simulink model "LCL_Inverter_Template"  (R2017a)
settings: Solver=ode4  StartTime=0.0  StopTime=0.04  FixedStep=1e-7  MaxStep=1e-7  AbsTol=1e-9
InitFcn:
  | clc;
  | clear all;
  | 
  | Ts_Control = 1e-4;
  | Ts_Pw = 1e-7;
  | T_dead = 30 * Ts_Pw;
  | 
  | fg=50;
  | Ed=360;
  | 
  | Kd = 0.12 ;
  | 
  | Kp = 0.067 ;
  | Ki = 330 ;
  | 
  | Apt_Carrier = 3 ;
  | 
  | C = 10e-6;
  | R =  0.05 ;
  | L1 = 600e-6 ;
  | R1 =  0.05 ;
  | L2 = 150e-6 ;
  | R2 =  0.05 ;
undefined symbols (not defined in the file or in its folder): DiscIntNeverNeededParam
libraries: powerlib x12, simulink x3, powerlib_extras x2, powerlib_meascontrol x2
settings Model: Creator=Administrator  LastModifiedBy=donghao
settings SolverCC: ZeroCrossControl=DisableAll
settings DataIOCC: LimitDataPoints=on  SaveFormat=Array  SignalLoggingSaveFormat=ModelDataLogs
settings OptimizationCC: ExpressionDepthLimit=2147483647  InitFltsAndDblsToZero=on  LifeSpan=inf
settings DebuggingCC: SaveWithParameterizedLinksMsg=none  UnderspecifiedInitializationDetection=Classic  MergeDetectMultiDrivingBlocksExec=none  SignalResolutionControl=TryResolveAllWithWarning  SolverPrmCheckMsg=warning  MultiTaskDSMMsg=warning  MultiTaskCondExecSysMsg=none  FcnCallInpInsideContextMsg=warning  UnconnectedInputMsg=none  UnconnectedOutputMsg=none  UnconnectedLineMsg=none  AllowSymbolicDim=off  StateNameClashWarn=warning  SFUnexpectedBacktrackingDiag=warning  SFNoUnconditionalDefaultTransitionDiag=warning  SFExecutionAtInitializationDiag=none
settings HardwareCC: ProdBitPerPointer=32  ProdBitPerSizeT=32  ProdBitPerPtrDiffT=32  ProdLargestAtomicFloat=None  ProdIntDivRoundTo=Undefined  ProdEndianess=Unspecified  ProdWordSize=32  ProdHWDeviceType=32-bit Generic
settings ModelReferenceCC: PropagateSignalLabelsOutOfModel=off
settings SFSimCC: SimParseCustomCode=off
settings GRTTargetCC: TargetFcnLib=ansi_tfl_tmw.mat  TargetLangStandard=C89/C90 (ANSI)  GeneratePreprocessorConditionals=Disable all  CombineOutputUpdateFcns=off  GRTInterface=on
settings ConfigComp: CovMetricSettings=dw  CovHtmlReporting=on  CovSaveCumulativeToWorkspaceVar=on  CovSaveSingleToWorkspaceVar=on  CovExternalEMLEnable=off

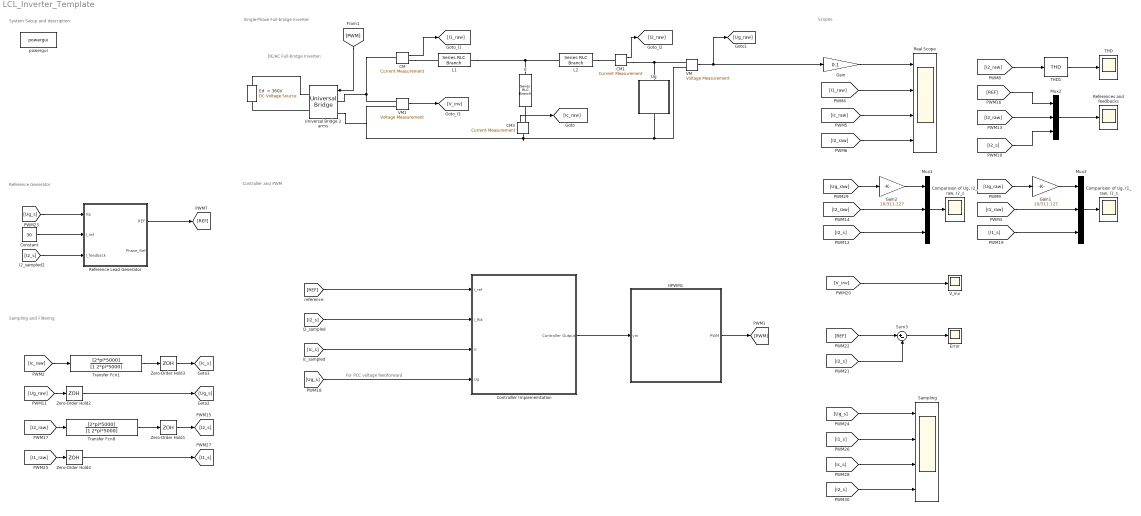
== system LCL_Inverter_Template ==
  note: For PCC voltage feedforward
  note: Sampling and Filtering
  note: System Setup and description:
  note: Single-Phase Full-bridge Inverter
  note: Scopes
  note: Controller and PWM
  note: DC/AC Full-bridge Inverter:
  note: Reference Generator
  C : powerlib/Elements/Series RLC Branch  LConnTagsString=__new0  RConnTagsString=__new0  BranchType=RC  Resistance=R  Inductance=0  SetiL0=off  InitialCurrent=0  Capacitance=C  Setx0=off  InitialVoltage=0  Measurements=None
  CM : powerlib/Measurements/Current Measurement  PhasorSimulation=off  OutputType=Complex  PSBequivalent=0
  CM1 : powerlib/Measurements/Current Measurement  PhasorSimulation=off  OutputType=Complex  PSBequivalent=0
  CM3 : powerlib/Measurements/Current Measurement  PhasorSimulation=off  OutputType=Complex  PSBequivalent=0
  "Comparision of Ug, I1_raw, I1_s" : Scope
  "Comparision of Ug, I2_raw, I2_s" : Scope
  Constant : Constant  Value=30
  Controlller Implememtation : Subsystem
  "Ed  = 360V  " : powerlib/Electrical Sources/DC Voltage Source  Description=source block  Amplitude=Ed  Measurements=None
      settings: AttributesFormatString=\n
  Error : Scope
  Gain : Gain  Gain=0.1
  Gain1 : Gain  Gain=10/311.127
  Gain2 : Gain  Gain=10/311.127
  HPWM1 : Subsystem
  L1 : powerlib/Elements/Series RLC Branch  LConnTagsString=__new0  RConnTagsString=__new0  BranchType=RL  Resistance=R1  Inductance=L1  SetiL0=off  InitialCurrent=0  Capacitance=1e-6  Setx0=off  InitialVoltage=0  Measurements=None
  L2 : powerlib/Elements/Series RLC Branch  LConnTagsString=__new0  RConnTagsString=__new0  BranchType=RL  Resistance=R2  Inductance=L2  SetiL0=off  InitialCurrent=0  Capacitance=1e-6  Setx0=off  InitialVoltage=0  Measurements=None
  Mux1 : Mux  Inputs=3
  Mux2 : Mux  Inputs=3
  Mux3 : Mux  Inputs=3
  Real Scope : Scope  NumInputPorts=4
  Reference Lead Generator : Subsystem
  References and feedbacks : Scope
  Sampling : Scope  NumInputPorts=4
  Sum3 : Sum  Inputs=|+-
  THD : Scope
  THD1 : powerlib_meascontrol/Measurements/THD  Freq=50  Ts=Ts_Pw
  Transfer Fcn1 : TransferFcn  Numerator=[2*pi*5000]  Denominator=[1 2*pi*5000]
  Transfer Fcn8 : TransferFcn  Numerator=[2*pi*5000]  Denominator=[1 2*pi*5000]
  Ug : Subsystem
  Universal Bridge 2 arms : powerlib/Power Electronics/Universal Bridge  Arms=2  SnubberResistance=1e3  SnubberCapacitance=1e-6  Device=IGBT / Diodes  Ron=1e-4  Lon=0  ForwardVoltages="[  1  1  ]"  ForwardVoltage=.8  GTOparameters=[ 10e-6 , 20e-6 ]  IGBTparameters=[ 1e-6 , 2e-6 ]  Measurements=None  Measurements_2=None  converterType=Rectifier
  VM : powerlib/Measurements/Voltage Measurement  PhasorSimulation=off  OutputType=Complex  PSBequivalent=0
  VM1 : powerlib/Measurements/Voltage Measurement  PhasorSimulation=off  OutputType=Complex  PSBequivalent=0
  V_inv : Scope
  Zero-Order Hold{1..4} (4 alike) : ZeroOrderHold  SampleTime=Ts_Control
  powergui : powerlib/powergui  SimulationMode=Discrete  SampleTime=Ts_Pw  frequency=60  Iterations=50  frequencyindice=50  Pbase=100e6  ErrMax=1e-4  UnitsV=kV  UnitsW=MW  buscounter=0  FunctionMessages=off  echomessages=off  EnableUseOfTLC=off  CurrentSourceSwitches=off  DisableSnubberDevices=off  DisableRonSwitches=off  DisableVfSwitches=off  DisplayEquations=off  SolverType=Tustin/Backward Euler (TBE)  Interpol=off  ExternalGateDelay=off  methode=off  Ts=0  x0status=blocks  SPID=off  SwTol=0  HookPort=off  RestoreLinks=warning  ResistiveCurrentMeasurement=off  Frange=[0:2:500]  Ylog=off  Xlog=on  ShowGrid=off  save=off  variable=ZData  structure=UGandIG1  ZoomFFT=off  StartTime=0.04  cycles=1  DisplayStyle=1  fundamental=50  FreqAxis=on  MaxFrequency=2000  frequencyindicesteady=1  RmsSteady=1  display=off
  wires:
  HPWM1/1(PWM) -> [PWM]
  VM/1 -> Gain/1, [Ug_raw]
  CM1/1 -> [I2_raw]
  Gain/1 -> Real Scope/1
  [I1_raw] -> Real Scope/2
  [Ic_raw] -> Real Scope/3
  [I2_raw] -> Real Scope/4
  Mux3/1 -> "Comparision of Ug, I1_raw, I1_s"/1
  [I1_raw] -> Mux3/2
  [Ug_raw] -> Gain1/1
  Gain1/1 -> Mux3/1
  [REF] -> Mux2/1
  Mux2/1 -> References and feedbacks/1
  [PWM] -> Universal Bridge 2 arms/1
  [I2_raw] -> THD1/1
  THD1/1 -> THD/1
  [I2_raw] -> Mux2/2
  CM3/1 -> [Ic_raw]
  CM/1 -> [I1_raw]
  Zero-Order Hold1/1 -> [I2_s]
  [I2_s] -> Controlller Implememtation/2(I_fbk)
  VM1/1 -> [V_inv]
  [V_inv] -> V_inv/1
  Reference Lead Generator/1(REF) -> [REF]
  [REF] -> Sum3/1
  [I2_s] -> Sum3/2
  Sum3/1 -> Error/1
  [Ug_s] -> Reference Lead Generator/1(Ug)
  [Ic_s] -> Controlller Implememtation/3(Ic)
  [Ug_s] -> Controlller Implememtation/4(Ug)
  Controlller Implememtation/1(Controller Output) -> HPWM1/1(vm)
  [Ug_raw] -> Zero-Order Hold2/1
  [REF] -> Controlller Implememtation/1(I_ref)
  Zero-Order Hold2/1 -> [Ug_s]
  Zero-Order Hold3/1 -> [Ic_s]
  [I2_s] -> Mux2/3
  [I1_s] -> Mux3/3
  [I1_raw] -> Zero-Order Hold4/1
  Zero-Order Hold4/1 -> [I1_s]
  [I2_s] -> Mux1/3
  [I2_raw] -> Mux1/2
  Gain2/1 -> Mux1/1
  [Ug_raw] -> Gain2/1
  Mux1/1 -> "Comparision of Ug, I2_raw, I2_s"/1
  [I2_s] -> Reference Lead Generator/3(I_feedback)
  Constant/1 -> Reference Lead Generator/2(I_ref)
  [I2_raw] -> Transfer Fcn8/1
  [Ug_s] -> Sampling/1
  [I1_s] -> Sampling/2
  [Ic_s] -> Sampling/3
  [I2_s] -> Sampling/4
  [Ic_raw] -> Transfer Fcn1/1
  Transfer Fcn8/1 -> Zero-Order Hold1/1
  Transfer Fcn1/1 -> Zero-Order Hold3/1
  connections:
  Universal Bridge 2 arms/RConn2 -- "Ed  = 360V  "/LConn1
  CM1/RConn1 -- VM/LConn1 -- Ug/RConn1
  L1/RConn1 -- L2/LConn1 -- C/LConn1
  CM/RConn1 -- L1/LConn1
  L2/RConn1 -- CM1/LConn1
  "Ed  = 360V  "/RConn1 -- Universal Bridge 2 arms/RConn1
  CM3/RConn1 -- C/RConn1
  VM1/LConn1 -- Universal Bridge 2 arms/LConn1 -- CM/LConn1
  Ug/LConn1 -- Universal Bridge 2 arms/LConn2 -- VM1/LConn2 -- CM3/LConn1 -- VM/LConn2

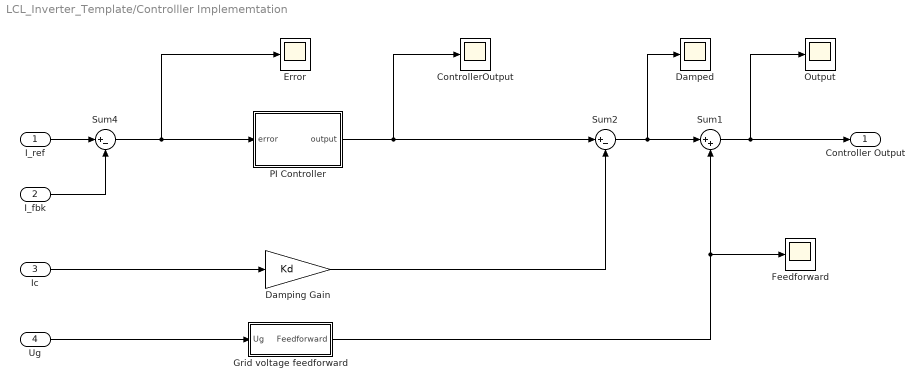
== system LCL_Inverter_Template/Controlller Implememtation ==
  I_ref : Inport
  I_fbk : Inport  Port=2
  Ic : Inport  Port=3
  Ug : Inport  Port=4
  ControllerOutput : Scope
  Damped : Scope
  Damping Gain : Gain  Gain=Kd
  Error : Scope
  Feedforward : Scope
  Grid voltage feedforward : Subsystem
  Output : Scope
  PI Controller : Subsystem
  Sum1 : Sum  Inputs=|++
  Sum2 : Sum  Inputs=|+-
  Sum4 : Sum  Inputs=|+-
  Controller Output : Outport
  wires:
  Ug/1 -> Grid voltage feedforward/1(Ug)
  Ic/1 -> Damping Gain/1
  PI Controller/1(output) -> Sum2/1, ControllerOutput/1
  Grid voltage feedforward/1(Feedforward) -> Feedforward/1, Sum1/2
  Sum1/1 -> Controller Output/1, Output/1
  Sum2/1 -> Sum1/1, Damped/1
  I_ref/1 -> Sum4/1
  I_fbk/1 -> Sum4/2
  Sum4/1 -> Error/1, PI Controller/1(error)
  Damping Gain/1 -> Sum2/2

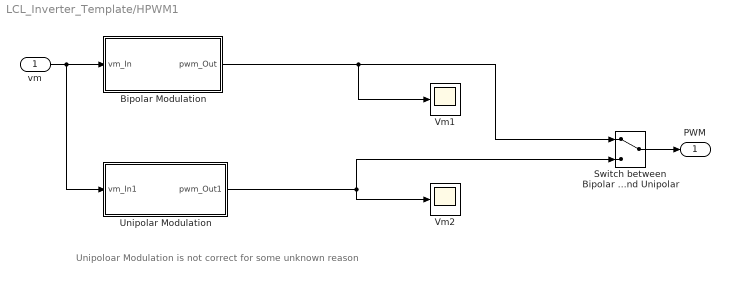
== system LCL_Inverter_Template/HPWM1 ==
  note: Unipoloar Modulation is not correct for some unknown reason
  vm : Inport
  Bipolar Modulation : Subsystem
  "Switch between Bipolar and Unipolar " : ManualSwitch
  Unipolar Modulation : Subsystem
  Vm1 : Scope
  Vm2 : Scope
  PWM : Outport
  wires:
  Bipolar Modulation/1(pwm_Out) -> "Switch between Bipolar and Unipolar "/1, Vm1/1
  vm/1 -> Unipolar Modulation/1(vm_In1), Bipolar Modulation/1(vm_In)
  "Switch between Bipolar and Unipolar "/1 -> PWM/1
  Unipolar Modulation/1(pwm_Out1) -> Vm2/1, "Switch between Bipolar and Unipolar "/2

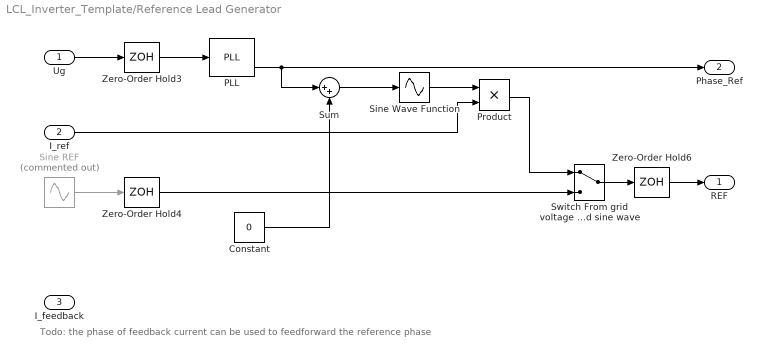
== system LCL_Inverter_Template/Reference Lead Generator ==
  note: Todo: the phase of feedback current can be used to feedforward the reference phase
  Ug : Inport
  I_ref : Inport  Port=2
  I_feedback : Inport  Port=3
  Constant : Constant  Value=0
  PLL : powerlib_meascontrol/PLL/PLL  Fmin=45  Par_Init=[0, 50]  ParK=[180, 3200, 1]  TcD=Ts_Control  MaxRateChangeFreq=12  FilterCutOffFreq=25  Ts=0  AGC=on
      settings: SourceProductName=Simscape Power Systems  SourceProductBaseCode=PS
  Product : Product
  Sine REF : Sin  Commented=on  Amplitude=40  Frequency=2*pi*fg  Phase=((2*pi)/360)*0  SampleTime=Ts_Pw
  Sine Wave Function : Sin  TimeSource=Use external signal  SampleTime=0
  Sum : Sum  Inputs=|++
  Switch From grid voltage phase or standard sine wave : ManualSwitch
  Zero-Order Hold3 : ZeroOrderHold  SampleTime=Ts_Control/2
  Zero-Order Hold4 : ZeroOrderHold  SampleTime=Ts_Control/2
  Zero-Order Hold6 : ZeroOrderHold  SampleTime=Ts_Control
  REF : Outport
  Phase_Ref : Outport  Port=2
  wires:
  Sine REF/1 -> Zero-Order Hold4/1
  Zero-Order Hold3/1 -> PLL/1
  Ug/1 -> Zero-Order Hold3/1
  Sine Wave Function/1 -> Product/1
  Switch From grid voltage phase or standard sine wave/1 -> Zero-Order Hold6/1
  Zero-Order Hold4/1 -> Switch From grid voltage phase or standard sine wave/2
  Product/1 -> Switch From grid voltage phase or standard sine wave/1
  PLL/2 -> Sum/1, Phase_Ref/1
  Sum/1 -> Sine Wave Function/1
  I_ref/1 -> Product/2
  Zero-Order Hold6/1 -> REF/1
  Constant/1 -> Sum/2

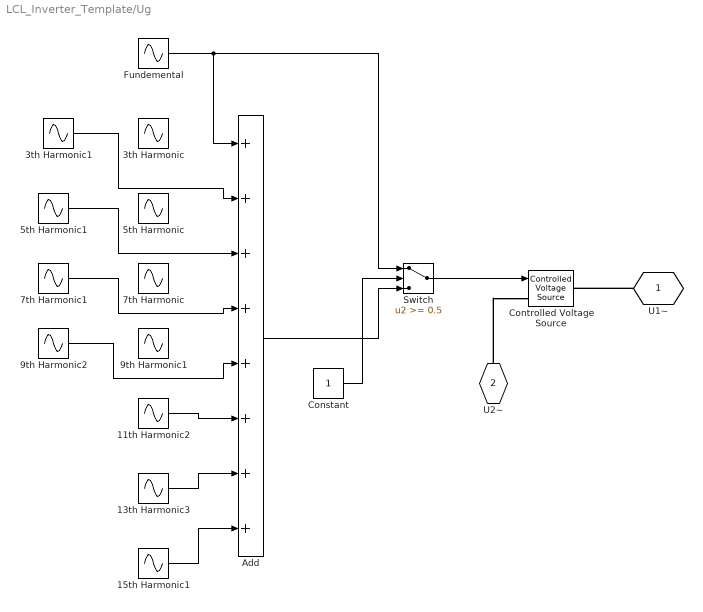
== system LCL_Inverter_Template/Ug ==
  11th Harmonic2 : Sin  Amplitude=sqrt(2)*220*0.0036  Frequency=2*pi*fg*11  Phase=2*pi*106/360  SampleTime=Ts_Pw
  13th Harmonic3 : Sin  Amplitude=sqrt(2)*220*0.0044  Frequency=2*pi*fg*13  SampleTime=Ts_Pw
  15th Harmonic1 : Sin  Amplitude=sqrt(2)*220*0.0049  Frequency=2*pi*fg*15  Phase=2*pi*44/360  SampleTime=Ts_Pw
  3th Harmonic : Sin  Amplitude=sqrt(2)*220*0.033*10  Frequency=2*pi*fg*3  SampleTime=Ts_Pw
  3th Harmonic1 : Sin  Amplitude=sqrt(2)*220*0.033  Frequency=2*pi*fg*3  SampleTime=Ts_Pw
  5th Harmonic : Sin  Amplitude=sqrt(2)*220*0.0043  Frequency=2*pi*fg*5  Phase=2*pi*178/360  SampleTime=Ts_Pw
  5th Harmonic1 : Sin  Amplitude=sqrt(2)*220*0.0043  Frequency=2*pi*fg*5  Phase=2*pi*178/360  SampleTime=Ts_Pw
  7th Harmonic : Sin  Amplitude=sqrt(2)*220*0.007*10  Frequency=2*pi*fg*7  Phase=2*pi*57/360  SampleTime=Ts_Pw
  7th Harmonic1 : Sin  Amplitude=sqrt(2)*220*0.007  Frequency=2*pi*fg*7  Phase=2*pi*57/360  SampleTime=Ts_Pw
  9th Harmonic1 : Sin  Amplitude=sqrt(2)*220*0.0061*10  Frequency=2*pi*fg*9  SampleTime=Ts_Pw
  9th Harmonic2 : Sin  Amplitude=sqrt(2)*220*0.0061  Frequency=2*pi*fg*9  SampleTime=Ts_Pw
  Add : Sum  Inputs=++++++++
  Constant : Constant  SampleTime=Ts_Pw
  Controlled Voltage Source : powerlib/Electrical Sources/Controlled Voltage Source  Initialize=on  Source_Type=AC  Amplitude=0  Phase=0  Frequency=50  Measurements=Voltage
  Fundemental : Sin  Amplitude=220*sqrt(2)  Frequency=2*pi*fg  SampleTime=Ts_Pw
  Switch : Switch  Threshold=0.5
  U1~ : PMIOPort  Port=1  Side=Right
  U2~ : PMIOPort  Port=2  Side=Left
  wires:
  Fundemental/1 -> Add/1, Switch/1
  Constant/1 -> Switch/2
  Add/1 -> Switch/3
  Switch/1 -> Controlled Voltage Source/1
  3th Harmonic1/1 -> Add/2
  5th Harmonic1/1 -> Add/3
  7th Harmonic1/1 -> Add/4
  9th Harmonic2/1 -> Add/5
  11th Harmonic2/1 -> Add/6
  13th Harmonic3/1 -> Add/7
  15th Harmonic1/1 -> Add/8
  connections:
  U1~/RConn1 -- Controlled Voltage Source/RConn1
  U2~/RConn1 -- Controlled Voltage Source/LConn1

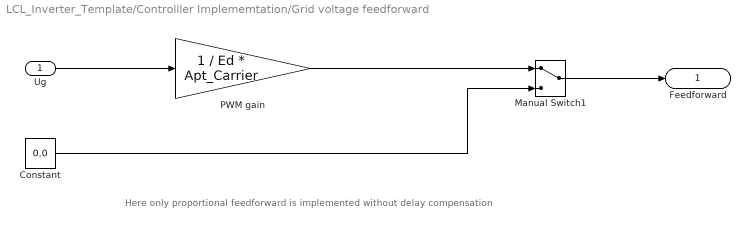
== system LCL_Inverter_Template/Controlller Implememtation/Grid voltage feedforward ==
  note: Here only proportional feedforward is implemented without delay compensation
  Ug : Inport
  Constant : Constant  Value=0.0
  Manual Switch1 : ManualSwitch
  PWM gain : Gain  Gain=1 / Ed * Apt_Carrier
  Feedforward : Outport
  wires:
  Ug/1 -> PWM gain/1
  Constant/1 -> Manual Switch1/2
  PWM gain/1 -> Manual Switch1/1
  Manual Switch1/1 -> Feedforward/1

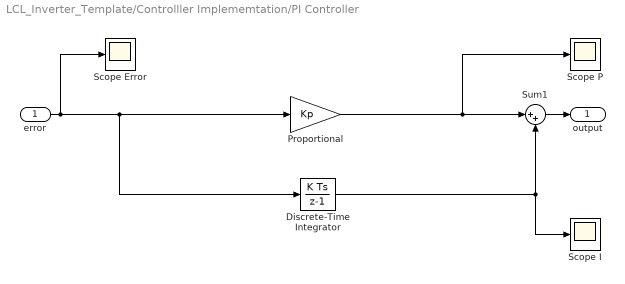
== system LCL_Inverter_Template/Controlller Implememtation/PI Controller ==
  error : Inport
  Discrete-Time Integrator : DiscreteIntegrator  gainval=Ki  InitialConditionSetting=State (most efficient)  SampleTime=Ts_Control  ICPrevOutput=DiscIntNeverNeededParam  ICPrevScaledInput=DiscIntNeverNeededParam
  Proportional : Gain  Gain=Kp
  Scope Error : Scope
  Scope I : Scope
  Scope P : Scope
  Sum1 : Sum  Inputs=|++
  output : Outport
  wires:
  Discrete-Time Integrator/1 -> Sum1/2, Scope I/1
  Sum1/1 -> output/1
  error/1 -> Scope Error/1, Discrete-Time Integrator/1, Proportional/1
  Proportional/1 -> Scope P/1, Sum1/1

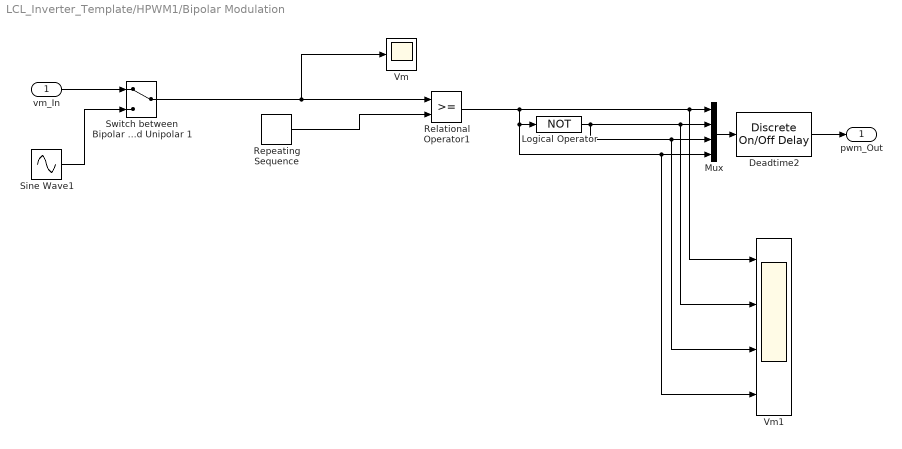
== system LCL_Inverter_Template/HPWM1/Bipolar Modulation ==
  vm_In : Inport
  Deadtime2 : powerlib_extras/Discrete  Control Blocks/Discrete On//Off Delay  type_delay=On delay  delay=T_dead  ic=0  Ts=Ts_Pw
  Logical Operator : Logic  Operator=NOT  AllPortsSameDT=off  OutDataTypeStr=boolean
  Mux : Mux
  Relational Operator1 : RelationalOperator  OutDataTypeStr=boolean  RndMeth=Nearest
  Repeating Sequence : simulink/Sources/Repeating Sequence  rep_seq_t="[0 Ts_Control/4  Ts_Control/2 Ts_Control*3/4 Ts_Control]"  rep_seq_y=[ Apt_Carrier 0 -Apt_Carrier 0 Apt_Carrier ]
  Sine Wave1 : Sin  Amplitude=2.5  Frequency=50 * 2 * pi  SampleTime=Ts_Control
  Switch between Bipolar and Unipolar 1 : ManualSwitch
  Vm : Scope
  Vm1 : Scope  NumInputPorts=4
  pwm_Out : Outport
  wires:
  Repeating Sequence/1 -> Relational Operator1/2
  Switch between Bipolar and Unipolar 1/1 -> Relational Operator1/1, Vm/1
  Deadtime2/1 -> pwm_Out/1
  Relational Operator1/1 -> Logical Operator/1, Vm1/4, Mux/4, Vm1/1, Mux/1
  Mux/1 -> Deadtime2/1
  Logical Operator/1 -> Vm1/2, Mux/2, Vm1/3, Mux/3
  vm_In/1 -> Switch between Bipolar and Unipolar 1/1
  Sine Wave1/1 -> Switch between Bipolar and Unipolar 1/2

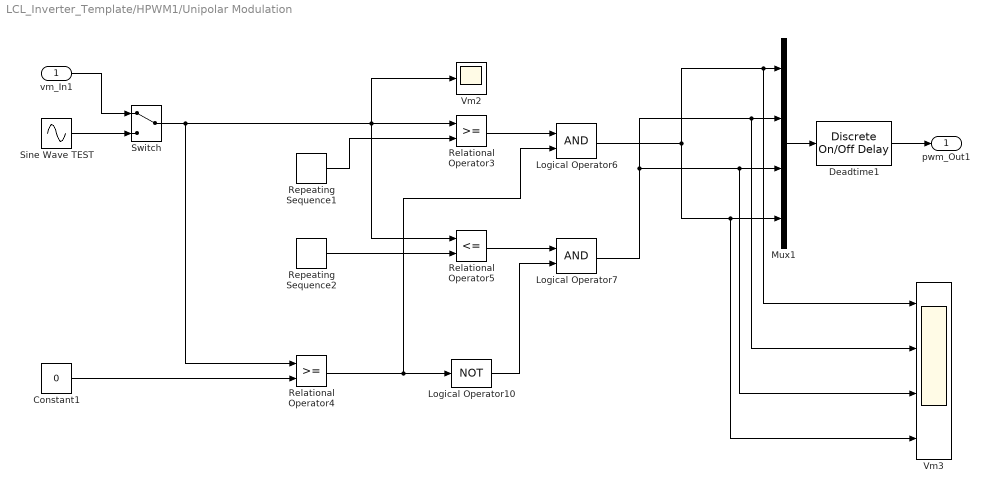
== system LCL_Inverter_Template/HPWM1/Unipolar Modulation ==
  vm_In1 : Inport
  Constant1 : Constant  Value=0
  Deadtime1 : powerlib_extras/Discrete  Control Blocks/Discrete On//Off Delay  type_delay=On delay  delay=T_dead  ic=0  Ts=Ts_Pw
  Logical Operator10 : Logic  Operator=NOT  AllPortsSameDT=off  OutDataTypeStr=boolean
  Logical Operator6 : Logic  AllPortsSameDT=off  OutDataTypeStr=boolean
  Logical Operator7 : Logic  AllPortsSameDT=off  OutDataTypeStr=boolean
  Mux1 : Mux
  Relational Operator3 : RelationalOperator  OutDataTypeStr=boolean  RndMeth=Nearest
  Relational Operator4 : RelationalOperator  OutDataTypeStr=boolean  RndMeth=Nearest
  Relational Operator5 : RelationalOperator  Operator=<=  OutDataTypeStr=boolean  RndMeth=Nearest
  Repeating Sequence1 : simulink/Sources/Repeating Sequence  rep_seq_t=[0 Ts_Control/2 Ts_Control]  rep_seq_y=[ Apt_Carrier 0 Apt_Carrier ]
  Repeating Sequence2 : simulink/Sources/Repeating Sequence  rep_seq_t=[0 Ts_Control/2 Ts_Control]  rep_seq_y=[ -Apt_Carrier 0 -Apt_Carrier ]
  Sine Wave TEST : Sin  Amplitude=2.5  Frequency=50 * 2 * pi  SampleTime=Ts_Control
  Switch : ManualSwitch
  Vm2 : Scope
  Vm3 : Scope  NumInputPorts=4
  pwm_Out1 : Outport
  wires:
  Deadtime1/1 -> pwm_Out1/1
  Repeating Sequence1/1 -> Relational Operator3/2
  Switch/1 -> Relational Operator5/1, Relational Operator3/1, Vm2/1, Relational Operator4/1
  Mux1/1 -> Deadtime1/1
  Sine Wave TEST/1 -> Switch/2
  Constant1/1 -> Relational Operator4/2
  vm_In1/1 -> Switch/1
  Relational Operator4/1 -> Logical Operator10/1, Logical Operator6/2
  Repeating Sequence2/1 -> Relational Operator5/2
  Relational Operator3/1 -> Logical Operator6/1
  Relational Operator5/1 -> Logical Operator7/1
  Logical Operator6/1 -> Vm3/1, Mux1/1, Vm3/4, Mux1/4
  Logical Operator10/1 -> Logical Operator7/2
  Logical Operator7/1 -> Vm3/3, Mux1/3, Vm3/2, Mux1/2
